simulink model "Lift"  (R2024b)
settings: Solver=VariableStepAuto  StartTime=0.0  StopTime=10.0  RelTol=1e-3
settings Model: Creator=Umesh Reddy K  LastModifiedBy=Umesh Reddy K

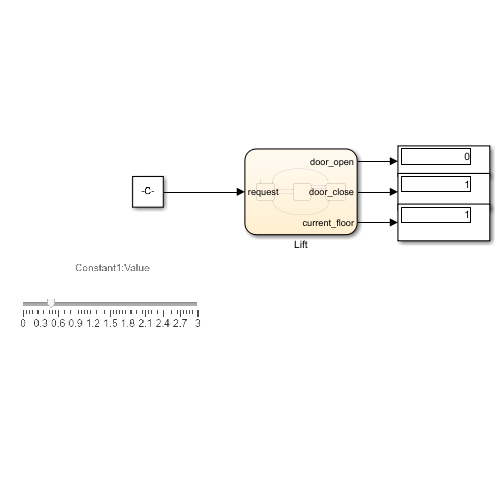
[thumbnail: Simulink's stored preview of the top-level diagram]
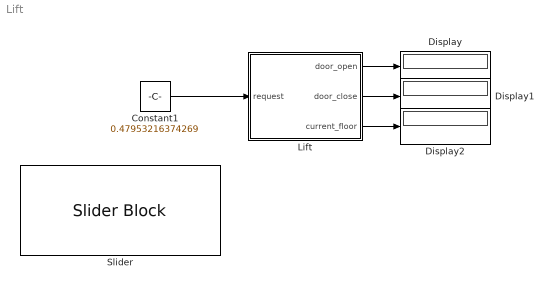
== system Lift ==
  Constant1 : Constant  Value=0.47953216374269
  Display : Display
  Display1 : Display
  Display2 : Display
  Lift : Stateflow chart  TreatAsAtomicUnit=on
  Slider : SliderBlock  ScaleMax=3
  wires:
  Constant1/1 -> Lift/1(request)
  Lift/1(door_open) -> Display/1
  Lift/2(door_close) -> Display1/1
  Lift/3(current_floor) -> Display2/1

== stateflow chart Lift/Lift ==
  state Floor1
    entry:
    door_open=true;
    current_floor = 1;
    after(10,sec);
    door_open=false;
    door_close=true;
  state Floor2
    entry:
    door_open=true;
    current_floor = 2;
    after(10,sec);
    door_open=false;
    door_close=true;
  state Floor3
    entry:
    door_open=true;
    current_floor = 3;
    after(10,sec);
    door_open=false;
    door_close=true;
  Floor3 -> Floor1 [order 2] : [request==1]
  (default) -> Floor1
  Floor2 -> Floor3 [order 2] : [request==3]
  Floor3 -> Floor2 [order 1] : [request==2]
  Floor1 -> Floor2 [order 1] : [request == 2]
  Floor2 -> Floor1 [order 1] : [request == 1]
  Floor1 -> Floor3 [order 2] : [request == 3]
  data: door_open output; door_close output; request input; current_floor output
